simulink model "model_simulink"  (R2024b)
settings: Solver=ode45  StartTime=0.0  StopTime=200  RelTol=1e-3
values from neighbouring files (symbols this model uses):
  MODEL = {}    [model.m]
undefined symbols (not defined in the file or in its folder): sigbuilder_block
settings Model: Creator=johne  LastModifiedBy=johne
settings SolverCC: MaxConsecutiveMinStep=10

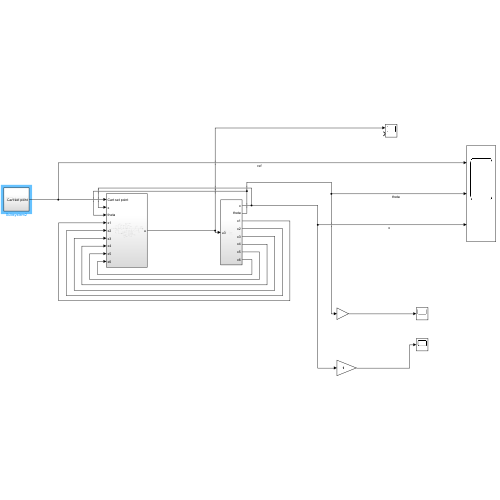
[thumbnail: Simulink's stored preview of the top-level diagram]
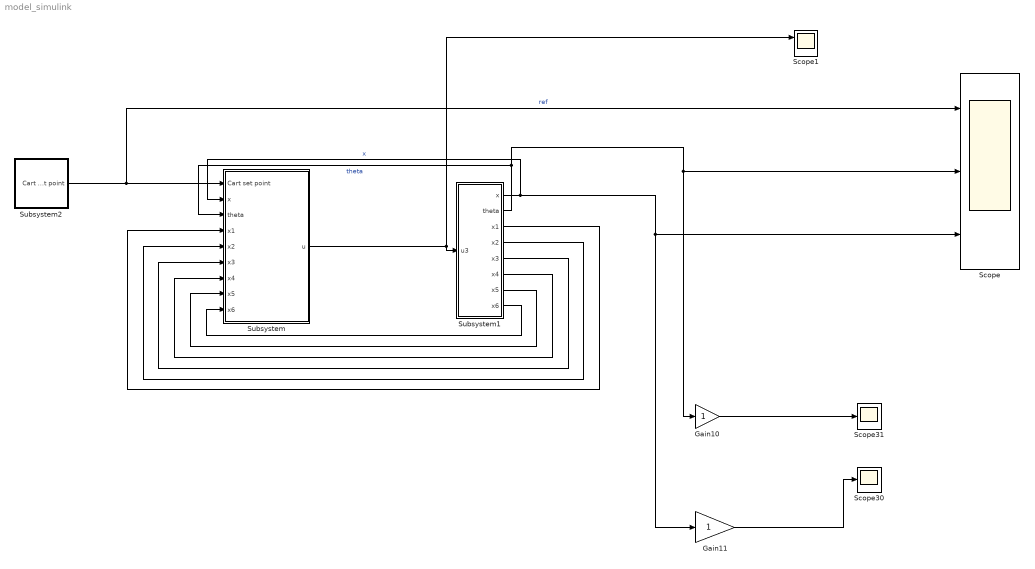
== system model_simulink ==
  Gain10 : Gain
  Gain11 : Gain
  Scope : Scope  NumInputPorts=3
  Scope1 : Scope  NumInputPorts=2
  Scope30 : Scope
  Scope31 : Scope
  Subsystem : Subsystem
  Subsystem1 : Subsystem
  Subsystem2 : Subsystem
  wires:
  Gain11/1 -> Scope30/1
  Gain10/1 -> Scope31/1
  Subsystem2/1(Cart set point) -> Scope/1, Subsystem/1(Cart set point)  "ref"
  Subsystem/1(u) -> Scope1/1, Subsystem1/1(u3)
  Subsystem1/1(x) -> Gain11/1, Scope/3, Subsystem/2(x)  "x"
  Subsystem1/2(theta) -> Gain10/1, Scope/2, Subsystem/3(theta)  "theta"
  Subsystem1/3(x1) -> Subsystem/4(x1)
  Subsystem1/4(x2) -> Subsystem/5(x2)
  Subsystem1/5(x3) -> Subsystem/6(x3)
  Subsystem1/6(x4) -> Subsystem/7(x4)
  Subsystem1/7(x5) -> Subsystem/8(x5)
  Subsystem1/8(x6) -> Subsystem/9(x6)

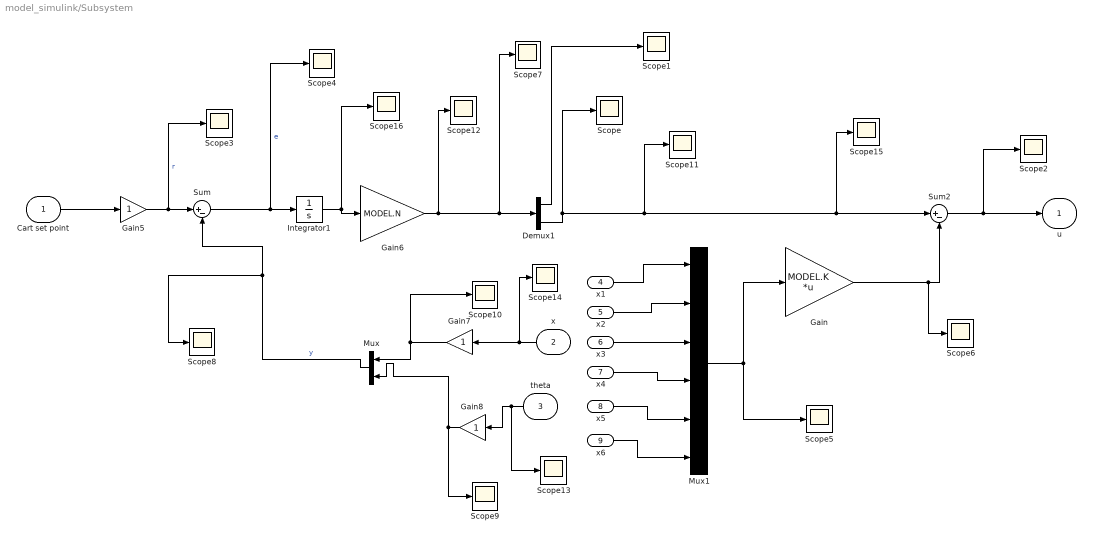
== system model_simulink/Subsystem ==
  Cart set point : Inport
  x : Inport  Port=2
  theta : Inport  Port=3
  x1 : Inport  Port=4
  x2 : Inport  Port=5
  x3 : Inport  Port=6
  x4 : Inport  Port=7
  x5 : Inport  Port=8
  x6 : Inport  Port=9
  Demux1 : Demux  Outputs=2
  Gain : Gain  Gain=MODEL.K  Multiplication=Matrix(K*u)
  Gain5 : Gain
  Gain6 : Gain  Gain=MODEL.N
  Gain7 : Gain
  Gain8 : Gain
  Integrator1 : Integrator
  Mux : Mux  Inputs=2
  Mux1 : Mux  Inputs=6
  Scope{,1..16} (17 alike) : Scope
  Sum : Sum  Inputs=|+-
  Sum2 : Sum  Inputs=|+-
  u : Outport  VectorParamsAs1DForOutWhenUnconnected=off
  wires:
  Sum/1 -> Integrator1/1, Scope4/1  "e"
  theta/1 -> Scope13/1, Gain8/1
  Gain5/1 -> Sum/1, Scope3/1  "r"
  x4/1 -> Mux1/4
  Gain7/1 -> Mux/1, Scope10/1
  Sum2/1 -> u/1, Scope2/1
  x/1 -> Scope14/1, Gain7/1
  x6/1 -> Mux1/6
  Gain/1 -> Scope6/1, Sum2/2
  Cart set point/1 -> Gain5/1
  Gain8/1 -> Mux/2, Scope9/1
  Mux1/1 -> Scope5/1, Gain/1
  Mux/1 -> Sum/2, Scope8/1  "y"
  x1/1 -> Mux1/1
  x3/1 -> Mux1/3
  x5/1 -> Mux1/5
  x2/1 -> Mux1/2
  Demux1/2 -> Scope15/1, Sum2/1, Scope11/1, Scope/1
  Demux1/1 -> Scope1/1
  Integrator1/1 -> Scope16/1, Gain6/1
  Gain6/1 -> Demux1/1, Scope7/1, Scope12/1

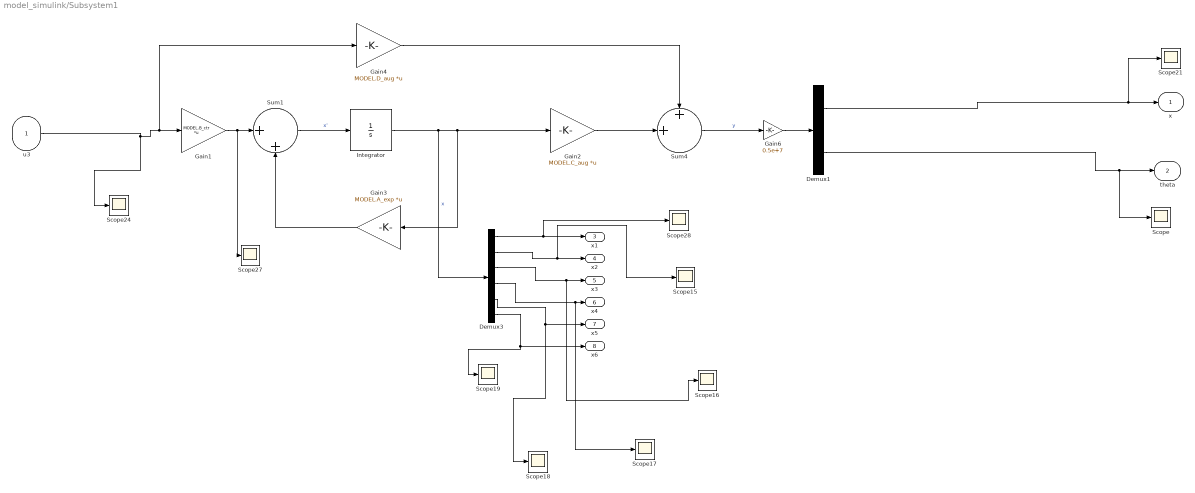
== system model_simulink/Subsystem1 ==
  u3 : Inport
  Demux1 : Demux  Outputs=2
  Demux3 : Demux  Outputs=6
  Gain1 : Gain  Gain=MODEL.B_ctr  Multiplication=Matrix(K*u)
  Gain2 : Gain  Gain=MODEL.C_aug  Multiplication=Matrix(K*u)
  Gain3 : Gain  Gain=MODEL.A_exp  Multiplication=Matrix(K*u)
  Gain4 : Gain  Gain=MODEL.D_aug  Multiplication=Matrix(K*u)
  Gain6 : Gain  Gain=0.5e+7
  Integrator : Integrator
  Scope{,15..19,21,24,27..28} (10 alike) : Scope
  Sum1 : Sum  Inputs=|++
  Sum4 : Sum  Inputs=++|
  x : Outport  VectorParamsAs1DForOutWhenUnconnected=off
  theta : Outport  Port=2  VectorParamsAs1DForOutWhenUnconnected=off
  x1 : Outport  Port=3
  x2 : Outport  Port=4
  x3 : Outport  Port=5
  x4 : Outport  Port=6
  x5 : Outport  Port=7
  x6 : Outport  Port=8
  wires:
  Sum4/1 -> Gain6/1  "y"
  Demux3/3 -> x3/1, Scope16/1
  Demux3/2 -> x2/1, Scope15/1
  Demux3/5 -> x5/1, Scope18/1
  Demux3/6 -> x6/1, Scope19/1
  Gain1/1 -> Scope27/1, Sum1/1
  Demux3/4 -> x4/1, Scope17/1
  u3/1 -> Scope24/1, Gain4/1, Gain1/1
  Gain4/1 -> Sum4/1
  Sum1/1 -> Integrator/1  "x'"
  Demux3/1 -> x1/1, Scope28/1
  Gain2/1 -> Sum4/2
  Gain3/1 -> Sum1/2
  Integrator/1 -> Demux3/1, Gain3/1, Gain2/1  "x"
  Demux1/1 -> Scope21/1, x/1
  Demux1/2 -> Scope/1, theta/1
  Gain6/1 -> Demux1/1

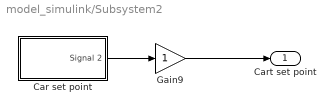
== system model_simulink/Subsystem2 ==
  Car set point : Subsystem  Tag=STV Subsys  LoadFcn=sigbuilder_block('load');  StartFcn=sigbuilder_block('start');  StopFcn=sigbuilder_block('stop');  ClipboardFcn=sigbuilder_block('clipboard');  mask(Sigbuilder block){tuvar=[0:10]}
      mask help: Simulink:masks:SigbuilderBlock_MD
      mask init:
      | if ~strcmp(get_param(bdroot(gcbh),'SimulationStatus'),'stopped') tuvar = sigbuilder_block('maskInit'); end
      settings: CopyFcn=sigbuilder_block('copy');  DeleteFcn=sigbuilder_block('delete');  ModelCloseFcn=sigbuilder_block('modelClose');  PreSaveFcn=sigbuilder_block('preSave');  PauseFcn=sigbuilder_block('pause');  ContinueFcn=sigbuilder_block('continue');  NameChangeFcn=sigbuilder_block('namechange');  OpenFcn=sigbuilder_block('open',[5.4 36 1141.2 516.6 ]);  CloseFcn=sigbuilder_block('close');
      mask Display: plot(0, 0, 100, 100,[2, 2, 32, 32, 2], [68, 8, 8, 68, 68],[32, 2], [38, 38], [32, 19, 2],[53, 60, 44], [32, 17, 17, 2],[16, 16, 31, 31]);txt = getActiveGroup(gcbh);text(2, 100, txt,'verticalAlignment', 'top');
  Gain9 : Gain
  Cart set point : Outport  VectorParamsAs1DForOutWhenUnconnected=off
  wires:
  Gain9/1 -> Cart set point/1
  Car set point/1(Signal 2) -> Gain9/1

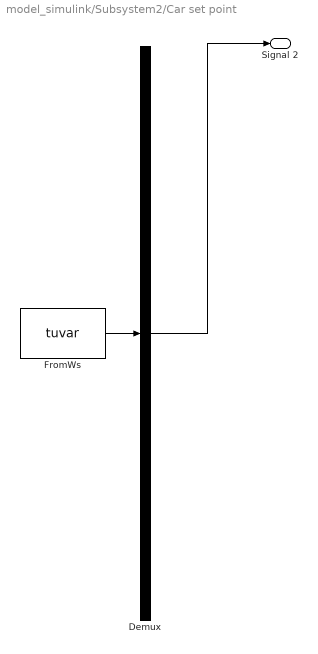
== system model_simulink/Subsystem2/Car set point ==
  Demux : Demux  Tag=STV Demux  Outputs=1
      settings: DisplayOption=none
  FromWs : FromWorkspace  Tag=STV FromWs  VariableName=tuvar
      SigBuilderData=|
      | common.afterFinalStr = 'Extrapolate'
      | common.sampleTime = 0
      | dataSet.timeRange = [0 200]
      | dataSet.name = 'Group 1'
      | sbobj.Groups.Name = 'Group 1'
      | sbobj.Groups.Signals.Name = 'Signal 2'
      | sbobj.Groups.Signals.XData = [0 6.6 6.6 22.2 22.2 53.8 53.8 88.4 88.4 109.2 109.2 134.8 134.8 161.8 161.8 182.8 182.8 200]
      | sbobj.Groups.Signals.YData = [0 0 0.8 0.8 -0.47 -0.47 0 0 0.51 0.51 0.685 0.685 -0.8 -0.8 0.51 0.51 0 0]
      | sbobj.Groups.TimeRange = [0 200]
  Signal 2 : Outport  Tag=STV Outport  VectorParamsAs1DForOutWhenUnconnected=off
  wires:
  FromWs/1 -> Demux/1
  Demux/1 -> Signal 2/1
